simulink model "Calibration_procedure"  (R2015a)
settings: Solver=FixedStepDiscrete  StartTime=0.0  StopTime=100  FixedStep=0.01  RelTol=1e-3
libraries: simulink x4, arduinolib x3
settings Model: ExtModeTrigDuration=2  Creator=pela  LastModifiedBy=Mattia
settings OptimizationCC: OptimizeModelRefInitCode=on  LifeSpan=1
settings DebuggingCC: UnderspecifiedInitializationDetection=Classic  MergeDetectMultiDrivingBlocksExec=none
settings HardwareCC: ProdBitPerInt=16  ProdBitPerPointer=8  ProdIntDivRoundTo=Zero  ProdEndianess=LittleEndian  ProdWordSize=8  ProdHWDeviceType=Atmel->AVR
settings RTWCC: SystemTargetFile=realtime.tlc  GenerateMakefile=off  TemplateMakefile=realtime.tmf  Description=Run on Target Hardware  RTWVerbose=off
settings ERTTargetCC: CombineOutputUpdateFcns=off  ExtModeTransport=3  ExtModeMexFile=ext_serial_win32_comm_rtt  ExtModeMexArgs=0 1 9600  ERTSrcFileBannerTemplate=realtime_code_template.cgt  ERTHdrFileBannerTemplate=realtime_code_template.cgt  ERTDataSrcFileTemplate=realtime_code_template.cgt  ERTDataHdrFileTemplate=realtime_code_template.cgt  ERTCustomFileTemplate=realtime_file_process.tlc

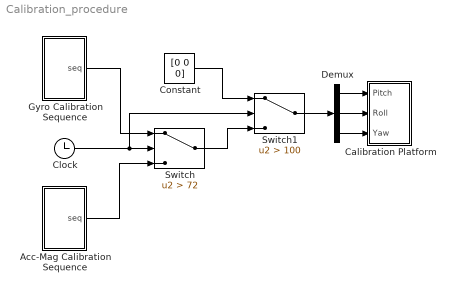
== system Calibration_procedure ==
  Acc-Mag Calibration Sequence : Subsystem
  Calibration Platform : Subsystem
  Clock : Clock
  Constant : Constant  Value=[0 0 0]
  Demux : Demux  Outputs=3
  Gyro Calibration Sequence : Subsystem
  Switch : Switch  Criteria=u2 > Threshold  Threshold=72
  Switch1 : Switch  Criteria=u2 > Threshold  Threshold=100
  wires:
  Demux/1 -> Calibration Platform/1(Pitch)
  Demux/2 -> Calibration Platform/2(Roll)
  Demux/3 -> Calibration Platform/3(Yaw)
  Clock/1 -> Switch1/2, Switch/2
  Gyro Calibration Sequence/1(seq) -> Switch/1
  Acc-Mag Calibration Sequence/1(seq) -> Switch/3
  Switch/1 -> Switch1/3
  Constant/1 -> Switch1/1
  Switch1/1 -> Demux/1

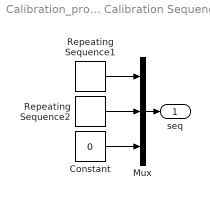
== system Calibration_procedure/Acc-Mag Calibration Sequence ==
  Constant : Constant  Value=0
  Mux : Mux  Inputs=3
  Repeating Sequence1 : simulink/Sources/Repeating Sequence  rep_seq_t=[0 1 2 3 4 5 6 7 8 9 10 11 12 13 14 15 16]  rep_seq_y=[-90 -90 -45 -45 0 0 45 45 90 90 45 45 0 0 -45 -45 -90]
  Repeating Sequence2 : simulink/Sources/Repeating Sequence  rep_seq_t=[0 7 8 (2*8-1) (2*8) (3*8-1) (3*8) (4*8-1) (4*8) (5*8-1) (5*8) (6*8-1) (6*8) (7*8-1) (7*8) (8*8-1) (8*8) (9*8)]  rep_seq_y=[180 180 135 135 90 90 45 45 0 0 -45 -45 -90 -90 -135 -135 -180 -180]
  seq : Outport
  wires:
  Repeating Sequence1/1 -> Mux/1
  Constant/1 -> Mux/3
  Repeating Sequence2/1 -> Mux/2
  Mux/1 -> seq/1

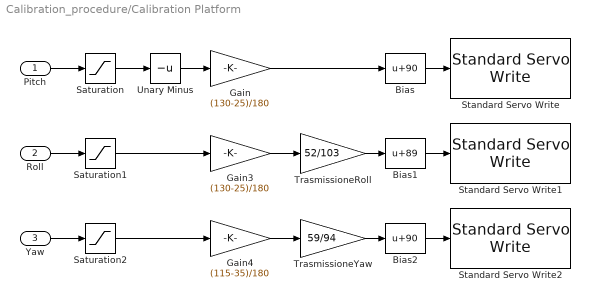
== system Calibration_procedure/Calibration Platform ==
  Pitch : Inport
  Roll : Inport  Port=2
  Yaw : Inport  Port=3
  Bias : Bias  Bias=90
  Bias1 : Bias  Bias=89
  Bias2 : Bias  Bias=90
  Gain : Gain  Gain=(130-25)/180
  Gain3 : Gain  Gain=(130-25)/180
  Gain4 : Gain  Gain=(115-35)/180
  Saturation : Saturate  UpperLimit=90  LowerLimit=-90
  Saturation1 : Saturate  UpperLimit=180  LowerLimit=-180
  Saturation2 : Saturate  UpperLimit=180  LowerLimit=-180
  Standard Servo Write : arduinolib/Standard Servo Write  pinNumber=9  blockPlatform=arduino
  Standard Servo Write1 : arduinolib/Standard Servo Write  pinNumber=10  blockPlatform=arduino
  Standard Servo Write2 : arduinolib/Standard Servo Write  pinNumber=11  blockPlatform=arduino
  TrasmissioneRoll : Gain  Gain=52/103
  TrasmissioneYaw : Gain  Gain=59/94
  Unary Minus : UnaryMinus
  wires:
  TrasmissioneRoll/1 -> Bias1/1
  Yaw/1 -> Saturation2/1
  TrasmissioneYaw/1 -> Bias2/1
  Saturation/1 -> Unary Minus/1
  Gain/1 -> Bias/1
  Bias1/1 -> Standard Servo Write1/1
  Bias/1 -> Standard Servo Write/1
  Bias2/1 -> Standard Servo Write2/1
  Gain3/1 -> TrasmissioneRoll/1
  Gain4/1 -> TrasmissioneYaw/1
  Roll/1 -> Saturation1/1
  Pitch/1 -> Saturation/1
  Unary Minus/1 -> Gain/1
  Saturation1/1 -> Gain3/1
  Saturation2/1 -> Gain4/1

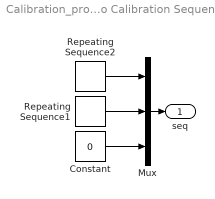
== system Calibration_procedure/Gyro Calibration Sequence ==
  Constant : Constant  Value=0
  Mux : Mux  Inputs=3
  Repeating Sequence1 : simulink/Sources/Repeating Sequence  rep_seq_t=[0 73 75 80 82 84 85 87 89 90 91 93 94 96 97 100]  rep_seq_y=[-180 -180 0 0 -90 -90 90 90 0 0 -90 -90 90 90 0 0]
  Repeating Sequence2 : simulink/Sources/Repeating Sequence  rep_seq_t=[0 76 77 78 79 90 91 96 97 100]  rep_seq_y=[90 90 -90 -90 0 0 90 90 0 0]
  seq : Outport
  wires:
  Mux/1 -> seq/1
  Repeating Sequence1/1 -> Mux/2
  Constant/1 -> Mux/3
  Repeating Sequence2/1 -> Mux/1
